simulink model "GenSync2_nosubsystem"  (R2014b)
settings: Solver=ode45  StartTime=0.0  StopTime=10.0  RelTol=1e-3
values from neighbouring files (symbols this model uses):
  delta0 = double(delta)    [CalcSteady1.m]    (also in Main2.m)
  J = (1/2)*(H*S)/(ws^2)    (= 7029.15711519)    [CalcSteady1.m]    (also in CalcSteady2.m; Main.m = 3.75; Main2.m = 18500)
  Ld = 7e-3    (= 0.007)    [CalcSteady1.m]    (also in CalcSteady2.m; Main.m; Main2.m; SolverODE.m)
  Lf = 7.384e-3    (= 0.007384)    [CalcSteady1.m]    (also in CalcSteady2.m; Main.m; Main2.m; SolverODE.m)
  Lm = 6.656e-3    (= 0.006656)    [CalcSteady1.m]    (also in CalcSteady2.m; Main.m; Main2.m; SolverODE.m)
  Lq = 5.61e-3    (= 0.00561)    [CalcSteady1.m]    (also in CalcSteady2.m; Main.m; Main2.m; SolverODE.m)
  phi_D0 = double(phi_d)    [CalcSteady1.m]    (also in Main2.m)
  phi_F0 = double(phi_f)    [CalcSteady1.m]    (also in Main2.m)
  phi_Q0 = double(phi_q)    [CalcSteady1.m]    (also in Main2.m)
  Rf = 0.985e-3    (= 0.000985)    [CalcSteady1.m]    (also in CalcSteady2.m; Main.m; Main2.m; SolverODE.m)
  Rs = 1.6e-3    (= 0.0016)    [CalcSteady1.m]    (also in CalcSteady2.m; Main.m; Main2.m; SolverODE.m)
  Wm0 = double(ws)    [CalcSteady1.m]    (also in Main2.m)
  ws = 2*pi*50    (= 314.159265359)    [CalcSteady1.m]    (also in CalcSteady2.m; Main.m; Main2.m; SolverODE.m)
settings Model: Creator=Eduardo Montilva  LastModifiedBy=Eduardo Montilva

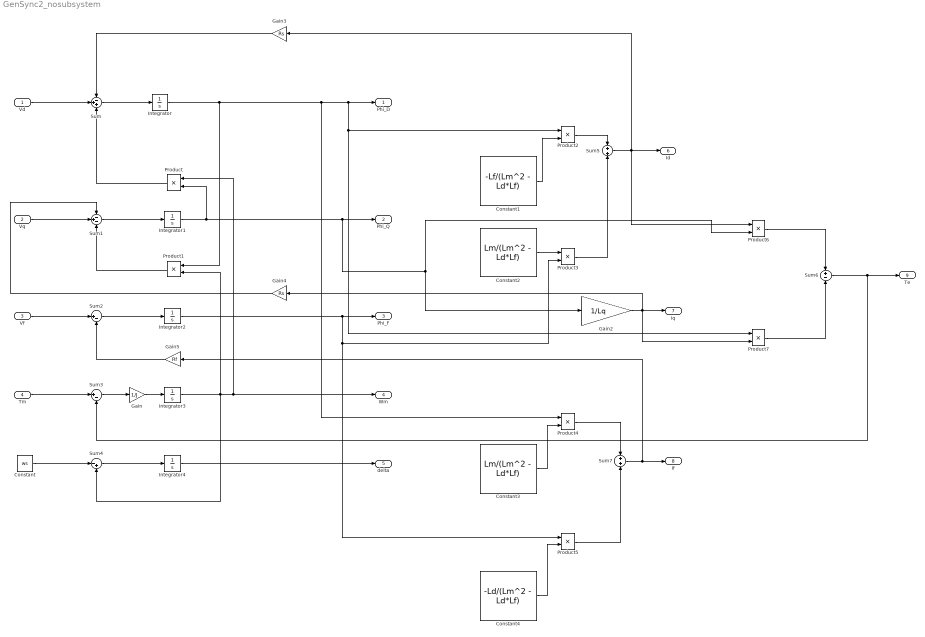
== system GenSync2_nosubsystem ==
  Vd : Inport
  Vq : Inport  Port=2
  Vf : Inport  Port=3
  Tm : Inport  Port=4
  Constant : Constant  Value=ws
  Constant1 : Constant  Value=-Lf/(Lm^2 - Ld*Lf)
  Constant2 : Constant  Value=Lm/(Lm^2 - Ld*Lf)
  Constant3 : Constant  Value=Lm/(Lm^2 - Ld*Lf)
  Constant4 : Constant  Value=-Ld/(Lm^2 - Ld*Lf)
  Gain : Gain  Gain=1/J
  Gain2 : Gain  Gain=1/Lq
  Gain3 : Gain  Gain=Rs
  Gain4 : Gain  Gain=Rs
  Gain5 : Gain  Gain=Rf
  Integrator : Integrator  InitialCondition=phi_D0
  Integrator1 : Integrator  InitialCondition=phi_Q0
  Integrator2 : Integrator  InitialCondition=phi_F0
  Integrator3 : Integrator  InitialCondition=Wm0
  Integrator4 : Integrator  InitialCondition=delta0
  Product{,1..7} (8 alike) : Product
  Sum : Sum  Inputs=-++
  Sum1 : Sum  Inputs=-+-
  Sum2 : Sum  Inputs=|+-
  Sum3 : Sum  Inputs=|+-
  Sum4 : Sum  Inputs=|-+
  Sum5 : Sum
  Sum6 : Sum  Inputs=+-
  Sum7 : Sum
  Phi_D : Outport
  Phi_Q : Outport  Port=2
  Phi_F : Outport  Port=3
  Wm : Outport  Port=4
  delta : Outport  Port=5
  Id : Outport  Port=6
  Iq : Outport  Port=7
  If : Outport  Port=8
  Te : Outport  Port=9
  wires:
  Sum7/1 -> If/1, Gain5/1
  Constant/1 -> Sum4/1
  Sum2/1 -> Integrator2/1
  Integrator2/1 -> Phi_F/1, Product5/1, Product3/2
  Vd/1 -> Sum/2
  Integrator4/1 -> delta/1
  Sum4/1 -> Integrator4/1
  Sum3/1 -> Gain/1
  Sum1/1 -> Integrator1/1
  Integrator1/1 -> Product/2, Phi_Q/1, Product6/2, Gain2/1
  Vq/1 -> Sum1/2
  Integrator3/1 -> Sum4/2, Product1/2, Wm/1, Product/1
  Gain/1 -> Integrator3/1
  Product/1 -> Sum/3
  Product3/1 -> Sum5/2
  Sum/1 -> Integrator/1
  Sum5/1 -> Id/1, Product6/1, Gain3/1
  Constant1/1 -> Product2/2
  Sum6/1 -> Te/1, Sum3/2
  Gain3/1 -> Sum/1
  Vf/1 -> Sum2/1
  Gain4/1 -> Sum1/1
  Gain5/1 -> Sum2/2
  Tm/1 -> Sum3/1
  Constant2/1 -> Product3/1
  Integrator/1 -> Product1/1, Product4/1, Phi_D/1, Product7/1, Product2/1
  Constant4/1 -> Product5/2
  Product4/1 -> Sum7/1
  Product7/1 -> Sum6/2
  Product5/1 -> Sum7/2
  Product6/1 -> Sum6/1
  Product2/1 -> Sum5/1
  Constant3/1 -> Product4/2
  Gain2/1 -> Iq/1, Product7/2, Gain4/1
  Product1/1 -> Sum1/3
